simulink model "Sim_3_observer_performance_no_noise"  (R2019b)
settings: Solver=VariableStepAuto  StartTime=0.0  StopTime=sim_time  FixedStep=0.01  MaxStep=0.1  MinStep=0.0001  RelTol=0.01  AbsTol=0.01
values from neighbouring files (symbols this model uses):
  Controller_Data = struct('K_p', K_p, 'K_v', K_v, 'K_i', K_i, 'M', M,     'D', D, 'U_ref', U_ref, 'mu', mu)    [Sim_10_init.m]    (also in Sim_11_init.m; Sim_12_init.m; Sim_3_4_and_5_init.m; Sim_7_8_userdef_init.m)
  D = [ 0.66  0    0 ... (first row only)    [Sim_10_init.m]    (also in Sim_11_init.m; Sim_12_init.m; Sim_3_4_and_5_init.m; Sim_7_8_userdef_init.m)
  K_p = 0.08*[1.1  0    0 ... (first row only)    [Sim_10_init.m]    (also in Sim_11_init.m; Sim_12_init.m; Sim_3_4_and_5_init.m; Sim_7_8_userdef_init.m)
  K_v = 1*[10   0       0 ... (first row only)    [Sim_10_init.m]    (also in Sim_11_init.m; Sim_12_init.m; Sim_3_4_and_5_init.m; Sim_7_8_userdef_init.m = 3*[10   0       0)
  LossOfSignalFalse = 1    [Sim_10_init.m]    (also in Sim_11_init.m; Sim_12_init.m; Sim_3_4_and_5_init.m; Sim_7_8_userdef_init.m)
  LossOfSignalTime = 10    [Sim_10_init.m]    (also in Sim_11_init.m; Sim_12_init.m; Sim_3_4_and_5_init.m = 30; Sim_7_8_userdef_init.m)
  LossOfSignalTrue = 0    [Sim_10_init.m]    (also in Sim_11_init.m; Sim_12_init.m; Sim_3_4_and_5_init.m; Sim_7_8_userdef_init.m)
  M = [ 16    0      0 ... (first row only)    [Sim_10_init.m]    (also in Sim_11_init.m; Sim_12_init.m; Sim_3_4_and_5_init.m; Sim_7_8_userdef_init.m)
  mu = 0.09    [Sim_10_init.m]    (also in Sim_11_init.m; Sim_12_init.m; Sim_3_4_and_5_init.m; Sim_7_8_userdef_init.m)
  Observergains = [L1, L2, L3]    [Sim_10_init.m]    (also in Sim_11_init.m; Sim_12_init.m; Sim_3_4_and_5_init.m; Sim_7_8_userdef_init.m)
  path_planner_data = [start_pos; end_pos; Radius; Center]    [Sim_10_init.m]    (also in Sim_11_init.m; Sim_12_init.m; Sim_3_4_and_5_init.m; Sim_7_8_userdef_init.m)
  pathparameter = 0    [Sim_10_init.m]    (also in Sim_11_init.m = 1; Sim_12_init.m; Sim_3_4_and_5_init.m = 1; Sim_7_8_userdef_init.m = 1)
  RegainOfSignalFalse = 0    [Sim_10_init.m]    (also in Sim_11_init.m; Sim_12_init.m; Sim_3_4_and_5_init.m; Sim_7_8_userdef_init.m)
  RegainOfSignalTime = 30    [Sim_10_init.m]    (also in Sim_11_init.m; Sim_12_init.m; Sim_3_4_and_5_init.m = 50; Sim_7_8_userdef_init.m)
  RegainOfSignalTrue = 1    [Sim_10_init.m]    (also in Sim_11_init.m; Sim_12_init.m; Sim_3_4_and_5_init.m; Sim_7_8_userdef_init.m)
  start_pos = [10; 20; pi/2 ]    [Sim_10_init.m]    (also in Sim_11_init.m = [0; 0; 0 ]; Sim_12_init.m = [0; 0; 0 ]; Sim_3_4_and_5_init.m = [0; 0; 0 ]; Sim_7_init.m = [0; 0; 0 ])
undefined symbols (not defined in the file or in its folder): tsamp, WP
(part 3 of 3)

== matlab function Sim_3_observer_performance_no_noise/Signal failure simulation, Dead reckoning function and Nonlinear Observer/Simlate a loss of signal function ==
  settings: updateMethod=DISCRETE
  data: eta_measured input size=3; eta_out output size=3; LossOfSignalValue output; Loss_of_signal_detection input; prior_measurement_in input; prior_measurement_out output
function [eta_out, LossOfSignalValue, prior_measurement_out] = SimLoS(eta_measured, Loss_of_signal_detection, prior_measurement_in)

% Simulates a loss of signal/frozen signal, where it keeps sending out the
% same measurement while the LossOfSignalDetection returns 0 as stated in
% task 4.4 and 4.5 from case B

    if not(Loss_of_signal_detection)
        eta_out = prior_measurement_in;
        prior_measurement_out = prior_measurement_in;
        LossOfSignalValue = Loss_of_signal_detection;
        
    else
        eta_out = eta_measured;
        prior_measurement_out = eta_measured;
        LossOfSignalValue = Loss_of_signal_detection;
    end
end

== matlab function Sim_3_observer_performance_no_noise/Controller/CtrlCustom_SLX/Backstepping controller/Sideslip compensation /LOS Lookahead Guidance ==
  data: p input; chi_d output size=1; WP input; segment_switch_lookahead_dist parameter; s input; track input; e_x output; e_y output
function [chi_d, e_x, e_y] = straight_line_path_handler(p, WP, segment_switch_lookahead_dist, s, track)

persistent current_segment;

if isempty(current_segment)
    current_segment = 1;
end

path_lookahead_dist = 0.5*segment_switch_lookahead_dist;

if not(track)
    p0 = WP(:,current_segment); % start wp in current segment
    p1 = WP(:, current_segment+1); % end wp in current segment
    num_segments = size(WP);
    num_segments = num_segments(2);

% update segment
% if next wp is closer to boat than path_lookahead_dist
% and not on last segment
    d_next_wp = p1 - p;
    d_next_wp = sqrt(dot(d_next_wp, d_next_wp));
    if current_segment + 1 < num_segments && d_next_wp <= segment_switch_lookahead_dist
        current_segment = current_segment + 1; 
        p0 = WP(:,current_segment);
        p1 = WP(:, current_segment+1);
    end
    % get path tangential angle
    % get x track and along track err
    alpha_k = atan2( p1(2) - p0(2), p1(1) - p0(1));
else
    % track
    p0 = WP(:,1); % start wp in current segment
    p1 = WP(:,2); % end wp in current segment
    alpha_k = atan2( p1(2) - p0(2), p1(1) - p0(1));
%     alpha_k
    p1(1) = p1(1) + s*3*cos(alpha_k);
    p1(2) = p1(2) + s*3*sin(alpha_k);
end

% current_segment = current_segment+1;
% cross track error
e_x = -(p(1) - p1(1))*sin(alpha_k) + (p(2) - p1(2))*cos(alpha_k);
% along track error
e_y = (p(1) - p1(1))*cos(alpha_k) + (p(2) - p1(2))*sin(alpha_k);
% lookahead based steering
chi_p = alpha_k;
%tan_chi_r = -e_x / path_lookahead_dist;
chi_r = atan(-e_x / path_lookahead_dist);
chi_d = chi_p + chi_r;

== matlab function Sim_3_observer_performance_no_noise/Controller/CtrlCustom_SLX/Backstepping controller/Sideslip compensation /Course calculation ==
  settings: updateMethod=DISCRETE
  data: p input; chi output size=1
function chi = compute_chi(p)

persistent p_prev;

if isempty(p_prev)
    p_prev = p;
    chi = 0;
else
    dy = p(2) - p_prev(2);
    dx = p(1) - p_prev(1);
    p_prev = p;
    chi = atan2(dy, dx);
    if chi < 0
        chi = chi + 2*pi;
    end
end

== matlab function Sim_3_observer_performance_no_noise/Controller/CtrlCustom_SLX/Backstepping controller/Sideslip compensation /MATLAB Function1 ==
  data: psi input; psi_ref input; psi_ref_new output
function psi_ref_new = ssa( psi, psi_ref)

val1 = psi_ref;
val2 = psi_ref + 2*pi;
val3 = psi_ref - 2*pi;

vals = [val1, val2, val3];

[m, i] = min(abs(vals - psi));

psi_ref_new = vals(i);

== matlab function Sim_3_observer_performance_no_noise/Controller/CtrlCustom_SLX/Transpose Rotation Matrix ==
  data: psi input; R_psi_trans output
function R_psi_trans = fcn(psi)
R_psi = [ cos(psi)  -sin(psi)   0  ;
                sin(psi)    cos(psi)  0  ; 
                    0              0         1  ] ;
                
R_psi_trans = transpose(R_psi);
end
